simulink model "Project_template_2b"  (R2014b)
settings: Solver=ode23tb  SolverMode=SingleTasking  StartTime=0.0  StopTime=600  RelTol=1e-6  AbsTol=1e-6
values from neighbouring files (symbols this model uses):
  a_0 = 0.6e-05    (= 6e-06)    [Project2B.m]
  A_max_wg = 0.02^2/4*pi    (= 0.000314159265359)    [Project2B.m]
  alpha_REF_manual = 0    [Project2B.m]
  Boost_control = 1    [Project2B.m]
  c_tc_fric = 1e-6    (= 1e-06)    [Project2B.m]
  Cd_wg = 0.9    [Project2B.m]
  dP_thrREF = 10e3    (= 10000)    [Project2B.m]
  J_tc = 1e-5    (= 1e-05)    [Project2B.m]
  KiDriver = 0.05    [Project2B.m]
  KpDriver = 0.8    [Project2B.m]
  KpThr = 1*10^-6    (= 1e-06)    [Project2B.m]
  KpWg = 10e-6    (= 1e-05)    [Project2B.m]
  N_e_manual = 1    [Project2B.m]
  N_e_step = 1    [Project2B.m]
  n_r = 2    [Project2B.m]
  NEND = NINI    (= 2500)    [Project2B.m]
  NeRampInit = 800    [Project2B.m]
  NeSlope = 1    [Project2B.m]
  NINI = 2500    [Project2B.m]
  pedEND = 1    [Project2B.m]
  pedINI = 0.0    (= 0)    [Project2B.m]
  pedPos_manual = 1    [Project2B.m]
  pedST = 30    [Project2B.m]
  T_es = mean(T_es)    [Project2B.m]
  T_ic = mean(T_ic)    [Project2B.m]
  tau_wg = 0.1    [Project2B.m]
  TiThr = 0.1    [Project2B.m]
  TiWg = 5    [Project2B.m]
  TqEvsNe =     [TqEvsNeMAP.mat]
  V_D = n_cyl*V_d    [Project2B.m]
  V_d = B^2/4*pi*s    [Project2B.m]
  V_ic = 10e-3    (= 0.01)    [Project2B.m]
  wg_REF_manual = 0    [Project2B.m]
undefined symbols (not defined in the file or in its folder): a_1, a_2, AFs, alphaEND, alphaINI, alphaST, BSRmax, C_2, C_d, c_fi, c_fr_0, C_P0, C_P1, c_r1, c_r2, cp_air, cp_exh, etaCmax, etaCmin, etaTmax, etaTmin, gamma_air, gamma_exh, k, k0, k1, K_I, K_p, n_0, n_1, n_2, n_cyl, n_ig_ch, NeST, Newton, p_amb, pCref, PiC_at_etaCmax, PsiMax, Q11, Q12, Q22, q_LHV, R_air, r_c, R_exh, Raphson, rComp, rho_air, rTurb, t_0, T_0, T_amb, T_hat_bef_thr, T_hat_im, tau_d_bc, tau_lambda, tau_th, TCref, V_em ... (+10)
libraries: simulink x1
(part 2 of 2)

== system Project_template_2b/Engine/m_dot_ac/n_vol ==
  p_im : Inport
  N : Inport  Port=2
  Constant : Constant  Value=n_0
  Gain : Gain  Gain=n_1
  Gain1 : Gain  Gain=n_2
  Sqrt : Sqrt  SaturateOnIntegerOverflow=on
  Sum of Elements : Sum  Inputs=+++
  n_vol : Outport
  wires:
  Sum of Elements/1 -> n_vol/1
  Constant/1 -> Sum of Elements/1
  p_im/1 -> Sqrt/1
  Sqrt/1 -> Gain/1
  Gain/1 -> Sum of Elements/2
  N/1 -> Gain1/1
  Gain1/1 -> Sum of Elements/3

== system Project_template_2b/ECU/Boost Control/Driver gas pedal interpretation/BMEP_ref -> p_im_ref ==
  In1 : Inport
  Add2 : Sum
  Constant2 : Constant  Value=C_P0
  Gain3 : Gain  Gain=1/C_P1
  Out1 : Outport
  wires:
  Constant2/1 -> Add2/2
  In1/1 -> Add2/1
  Gain3/1 -> Out1/1  "p_im_REF"
  Add2/1 -> Gain3/1

== system Project_template_2b/ECU/Boost Control/Throttle Feed Forward /A_eff_ref ==
  m_dot_air_ref : Inport
  Psi : Inport  Port=2
  p_ic : Inport  Port=3
  Divide1 : Product  Inputs=*/
  Divide2 : Product  Inputs=*/
  Gain : Gain  Gain=sqrt(R_air*T_ic)
  A_eff_ref : Outport
  wires:
  Psi/1 -> Divide1/2
  m_dot_air_ref/1 -> Divide1/1
  Divide1/1 -> Gain/1
  Gain/1 -> Divide2/1
  Divide2/1 -> A_eff_ref/1
  p_ic/1 -> Divide2/2

== system Project_template_2b/ECU/Boost Control/Throttle Feed Forward /Cylinder air flow REF ==
  p_im_REF : Inport
  N [rps] : Inport  Port=2
  Gain : Gain  Gain=n_cyl*V_d/(n_r*R_air*T_hat_im)
  Product : Product  Inputs=3
  Volymetrisk effektivitet : Subsystem
  m_dot_ac_REF : Outport
  wires:
  N [rps]/1 -> Product/3, Volymetrisk effektivitet/2(N)
  p_im_REF/1 -> Product/1, Volymetrisk effektivitet/1(" p_im")
  Product/1 -> Gain/1
  Gain/1 -> m_dot_ac_REF/1
  Volymetrisk effektivitet/1(eta_vol) -> Product/2

== system Project_template_2b/ECU/Boost Control/Throttle Feed Forward /Psi(PI) ==
  PI : Inport
  (g+1)/g : Constant  Value=(gamma_air+1)/gamma_air
  2/g : Constant  Value=2/gamma_air
  2g/(g-1) : Constant  Value=(2*gamma_air)/(gamma_air-1)
  DivZeroProtect : MinMax  Function=max  Inputs=2
  Math Function : Math  Operator=pow  SaturateOnIntegerOverflow=on
  Math Function1 : Math  Operator=pow  SaturateOnIntegerOverflow=on
  MinMax : MinMax  Function=max  Inputs=2
  PI critical (2/(g+1))^(g/(g-1)) : Constant  Value=(2/(gamma_air+1))^(gamma_air/(gamma_air-1))
  Product : Product  RndMeth=Zero
  Sqrt : Sqrt  AlgorithmType=Newton-Raphson  SaturateOnIntegerOverflow=on
  Subtract : Sum  Inputs=+-
  "[0,1]" : Saturate  UpperLimit=1  LowerLimit=0
  eps : Constant  Value=eps
  Psi : Outport
  wires:
  DivZeroProtect/1 -> Psi/1
  eps/1 -> DivZeroProtect/2
  Sqrt/1 -> DivZeroProtect/1  "Psi"
  Product/1 -> Sqrt/1
  2g/(g-1)/1 -> Product/2
  Subtract/1 -> Product/1
  Math Function1/1 -> Subtract/2
  Math Function/1 -> Subtract/1
  "[0,1]"/1 -> MinMax/1
  (g+1)/g/1 -> Math Function1/2
  2/g/1 -> Math Function/2
  MinMax/1 -> Math Function1/1, Math Function/1  "PIlim"
  PI critical (2/(g+1))^(g/(g-1))/1 -> MinMax/2
  PI/1 -> "[0,1]"/1  "PI"

== system Project_template_2b/ECU/Fuel Cont/Air cylinder/n_vol ==
  p_im : Inport
  N : Inport  Port=2
  Constant : Constant  Value=n_0
  Gain : Gain  Gain=n_1
  Gain1 : Gain  Gain=n_2
  Sqrt : Sqrt  SaturateOnIntegerOverflow=on
  Sum of Elements : Sum  Inputs=+++
  n_vol : Outport
  wires:
  Sum of Elements/1 -> n_vol/1
  Constant/1 -> Sum of Elements/1
  p_im/1 -> Sqrt/1
  Sqrt/1 -> Gain/1
  Gain/1 -> Sum of Elements/2
  N/1 -> Gain1/1
  Gain1/1 -> Sum of Elements/3

== system Project_template_2b/Engine/Cylinder/W_ig/eta_tilde_ig ==
  lambda_cyl : Inport
  Constant : Constant
  Gain : Gain  Gain=(1-1/r_c^(gamma_air-1))*n_ig_ch
  MinMax : MinMax  Inputs=2
  eta_tilde_ig : Outport
  wires:
  lambda_cyl/1 -> MinMax/1
  Constant/1 -> MinMax/2
  MinMax/1 -> Gain/1
  Gain/1 -> eta_tilde_ig/1

== system Project_template_2b/Engine/Turbocharger/Compressor/PiCmax ==
  Tamb : Inport
  w_tc : Inport  Port=2
  Add : Sum
  Constant : Constant
  Constant1 : Constant  Value=gamma_air/(gamma_air-1)
  Divide : Product  Inputs=*/
  Gain : Gain  Gain=rComp
  Gain1 : Gain  Gain=PsiMax/(2*cp_air)
  Math Function : Math  Operator=square  SaturateOnIntegerOverflow=on
  Math Function1 : Math  Operator=pow  SaturateOnIntegerOverflow=on
  PiCmax : Outport
  wires:
  Math Function1/1 -> PiCmax/1
  Tamb/1 -> Divide/2
  w_tc/1 -> Gain/1
  Gain/1 -> Math Function/1
  Math Function/1 -> Gain1/1
  Gain1/1 -> Divide/1
  Divide/1 -> Add/1
  Constant/1 -> Add/2
  Add/1 -> Math Function1/1
  Constant1/1 -> Math Function1/2

== system Project_template_2b/Engine/Turbocharger/Compressor/Tc ==
  etaC : Inport
  PiC : Inport  Port=2
  Tamb : Inport  Port=3
  Add : Sum  Inputs=+-
  Add1 : Sum
  Constant : Constant  Value=(gamma_air-1)/gamma_air
  Constant1 : Constant
  Divide : Product  Inputs=*/
  Math Function : Math  Operator=pow  SaturateOnIntegerOverflow=on
  Product : Product
  Tc : Outport
  wires:
  Add1/1 -> Tc/1
  PiC/1 -> Math Function/1
  etaC/1 -> Divide/2
  Tamb/1 -> Add1/2, Product/2
  Constant/1 -> Math Function/2
  Constant1/1 -> Add/2
  Math Function/1 -> Add/1
  Add/1 -> Divide/1
  Divide/1 -> Product/1
  Product/1 -> Add1/1

== system Project_template_2b/Engine/Turbocharger/Compressor/Tq_c ==
  Wc : Inport
  Tc : Inport  Port=2
  Tamb : Inport  Port=3
  w_tc : Inport  Port=4
  Add : Sum  Inputs=+-
  Divide : Product  Inputs=*/
  Gain : Gain  Gain=cp_air
  Product : Product
  Tq_c : Outport
  wires:
  w_tc/1 -> Divide/2
  Wc/1 -> Product/1
  Tc/1 -> Add/1
  Tamb/1 -> Add/2
  Add/1 -> Gain/1
  Gain/1 -> Product/2
  Product/1 -> Divide/1
  Divide/1 -> Tq_c/1

== system Project_template_2b/Engine/Turbocharger/Compressor/WcCorr2Wc ==
  p_amb : Inport
  T_amb : Inport  Port=2
  m_dot_cCorr : Inport  Port=3
  Constant : Constant  Value=0
  Divide : Product  Inputs=*/
  Gain : Gain  Gain=1/TCref
  Gain1 : Gain  Gain=1/pCref
  MinMax : MinMax  Function=max  Inputs=2
  Product : Product
  Sqrt : Sqrt  SaturateOnIntegerOverflow=on
  m_dot_c : Outport
  wires:
  m_dot_cCorr/1 -> Product/1
  p_amb/1 -> Gain1/1
  T_amb/1 -> Gain/1
  Product/1 -> m_dot_c/1
  Gain1/1 -> Divide/1
  Sqrt/1 -> Divide/2
  Divide/1 -> Product/2
  MinMax/1 -> Sqrt/1
  Gain/1 -> MinMax/1
  Constant/1 -> MinMax/2

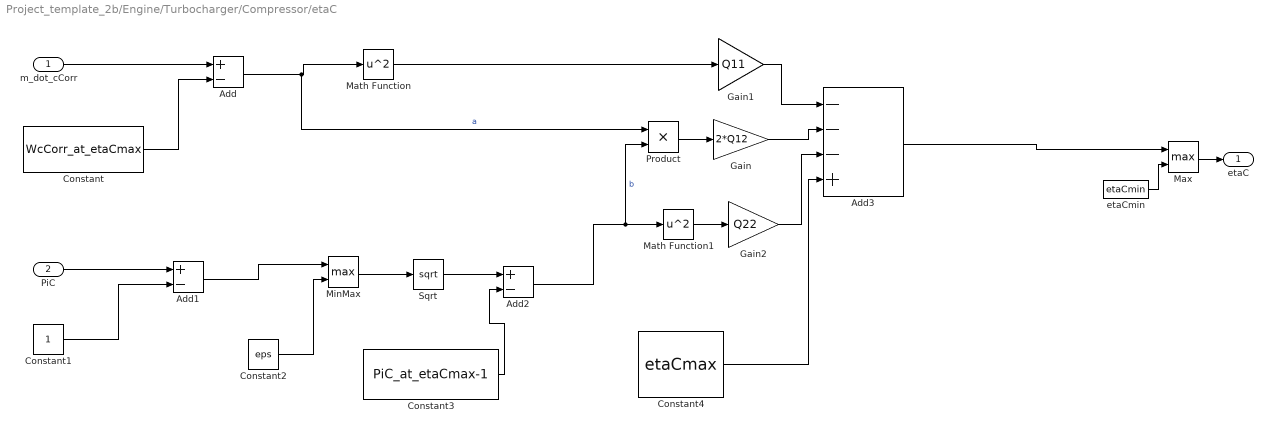
== system Project_template_2b/Engine/Turbocharger/Compressor/etaC ==
  m_dot_cCorr : Inport
  PiC : Inport  Port=2
  Add : Sum  Inputs=+-
  Add1 : Sum  Inputs=+-
  Add2 : Sum  Inputs=+-
  Add3 : Sum  Inputs=---+
  Constant : Constant  Value=WcCorr_at_etaCmax
  Constant1 : Constant
  Constant2 : Constant  Value=eps
  Constant3 : Constant  Value=PiC_at_etaCmax-1
  Constant4 : Constant  Value=etaCmax
  Gain : Gain  Gain=2*Q12
  Gain1 : Gain  Gain=Q11
  Gain2 : Gain  Gain=Q22
  Math Function : Math  Operator=square  SaturateOnIntegerOverflow=on
  Math Function1 : Math  Operator=square  SaturateOnIntegerOverflow=on
  Max : MinMax  Function=max  Inputs=2
  MinMax : MinMax  Function=max  Inputs=2
  Product : Product
  Sqrt : Sqrt  SaturateOnIntegerOverflow=on
  etaCmin : Constant  Value=etaCmin
  etaC : Outport
  wires:
  PiC/1 -> Add1/1
  m_dot_cCorr/1 -> Add/1
  Max/1 -> etaC/1
  etaCmin/1 -> Max/2
  Add3/1 -> Max/1
  Constant/1 -> Add/2
  Add/1 -> Product/1, Math Function/1  "a"
  Constant1/1 -> Add1/2
  Constant2/1 -> MinMax/2
  Add1/1 -> MinMax/1
  MinMax/1 -> Sqrt/1
  Sqrt/1 -> Add2/1
  Constant3/1 -> Add2/2
  Math Function/1 -> Gain1/1
  Gain1/1 -> Add3/1
  Gain/1 -> Add3/2
  Gain2/1 -> Add3/3
  Add2/1 -> Product/2, Math Function1/1  "b"
  Math Function1/1 -> Gain2/1
  Product/1 -> Gain/1
  Constant4/1 -> Add3/4

== system Project_template_2b/Engine/Turbocharger/Compressor/m_dot_cCorr ==
  PiCmax : Inport
  PiC : Inport  Port=2
  Add : Sum  Inputs=-+
  Constant : Constant
  Constant1 : Constant  Value=eps
  Divide : Product  Inputs=/*
  Gain : Gain  Gain=WcCorrMax
  Math Function : Math  Operator=square  SaturateOnIntegerOverflow=on
  MinMax : MinMax  Function=max  Inputs=2
  Sqrt : Sqrt  SaturateOnIntegerOverflow=on
  m_dot_cCorr : Outport
  wires:
  PiC/1 -> Divide/2
  PiCmax/1 -> Divide/1
  Gain/1 -> m_dot_cCorr/1  "m_dot_cCorr"
  Divide/1 -> Math Function/1
  Constant/1 -> Add/2
  Math Function/1 -> Add/1
  Sqrt/1 -> Gain/1
  MinMax/1 -> Sqrt/1
  Add/1 -> MinMax/1
  Constant1/1 -> MinMax/2

== system Project_template_2b/Engine/Turbocharger/Turbine/BSR ==
  T_em : Inport
  PiT : Inport  Port=2
  w_tc [rad/s] : Inport  Port=3
  Add : Sum  Inputs=-+
  Constant : Constant  Value=-(gamma_exh-1)/gamma_exh
  Constant1 : Constant
  Divide : Product  Inputs=*/
  Gain : Gain  Gain=2*cp_exh
  Gain1 : Gain  Gain=rTurb
  Math Function : Math  Operator=pow  SaturateOnIntegerOverflow=on
  Product : Product
  Sqrt : Sqrt  SaturateOnIntegerOverflow=on
  BSR : Outport
  wires:
  PiT/1 -> Math Function/1
  Constant/1 -> Math Function/2
  Math Function/1 -> Add/1
  Constant1/1 -> Add/2
  Add/1 -> Product/1
  T_em/1 -> Product/2
  Product/1 -> Gain/1
  Sqrt/1 -> Divide/2
  Gain1/1 -> Divide/1
  w_tc [rad/s]/1 -> Gain1/1
  Divide/1 -> BSR/1
  Gain/1 -> Sqrt/1

== system Project_template_2b/Engine/Turbocharger/Turbine/PiT ==
  p_em : Inport
  p_t : Inport  Port=2
  MinMax : MinMax  Function=max  Inputs=2
  Product4 : Product  Inputs=*/  RndMeth=Zero
  one1 : Constant
  PiT : Outport
  wires:
  p_t/1 -> Product4/2
  MinMax/1 -> PiT/1  "PiT"
  p_em/1 -> Product4/1
  one1/1 -> MinMax/2
  Product4/1 -> MinMax/1

== system Project_template_2b/Engine/Turbocharger/Turbine/TFP2Wt ==
  p_em [Pa] : Inport
  TFP : Inport  Port=2
  T_em : Inport  Port=3
  Constant1 : Constant  Value=1e-3
  Divide : Product  Inputs=*/
  Product : Product  Inputs=3
  Sqrt : Sqrt  SaturateOnIntegerOverflow=on
  Wt : Outport
  wires:
  Divide/1 -> Wt/1
  TFP/1 -> Product/1
  p_em [Pa]/1 -> Product/2
  Product/1 -> Divide/1
  T_em/1 -> Sqrt/1
  Sqrt/1 -> Divide/2
  Constant1/1 -> Product/3

== system Project_template_2b/Engine/Turbocharger/Turbine/TFPmod ==
  PiT : Inport
  Add : Sum  Inputs=-+
  Constant : Constant  Value=-k1
  Constant1 : Constant
  Constant2 : Constant  Value=eps
  Gain : Gain  Gain=k0
  Math Function : Math  Operator=pow  SaturateOnIntegerOverflow=on
  MinMax : MinMax  Function=max  Inputs=2
  Sqrt : Sqrt  SaturateOnIntegerOverflow=on
  TFPmod : Outport
  wires:
  PiT/1 -> Math Function/1
  Constant/1 -> Math Function/2
  Math Function/1 -> Add/1
  Constant1/1 -> Add/2
  Constant2/1 -> MinMax/2
  Add/1 -> MinMax/1
  MinMax/1 -> Sqrt/1
  Sqrt/1 -> Gain/1
  Gain/1 -> TFPmod/1

== system Project_template_2b/Engine/Turbocharger/Turbine/Tq_t ==
  Wt : Inport
  Tem : Inport  Port=2
  Tt : Inport  Port=3
  w_tc : Inport  Port=4
  Add : Sum  Inputs=+-
  Divide : Product  Inputs=*/
  Gain : Gain  Gain=cp_exh
  Product : Product
  Tq_t : Outport
  wires:
  Tt/1 -> Add/2
  Tem/1 -> Add/1
  Add/1 -> Gain/1
  Gain/1 -> Product/2
  Wt/1 -> Product/1
  w_tc/1 -> Divide/2
  Product/1 -> Divide/1
  Divide/1 -> Tq_t/1

== system Project_template_2b/Engine/Turbocharger/Turbine/Tt ==
  Tem : Inport
  etaT : Inport  Port=2
  PiT : Inport  Port=3
  Add : Sum  Inputs=-+
  Add1 : Sum  Inputs=+-
  Constant : Constant  Value=-(gamma_exh-1)/gamma_exh
  Constant1 : Constant
  Constant2 : Constant
  Math Function : Math  Operator=pow  SaturateOnIntegerOverflow=on
  Product : Product
  Product1 : Product
  Tt : Outport
  wires:
  PiT/1 -> Math Function/1
  Constant/1 -> Math Function/2
  Constant1/1 -> Add/2
  Add/1 -> Product/1
  etaT/1 -> Product1/2
  Tem/1 -> Product/2
  Product/1 -> Tt/1
  Product1/1 -> Add/1
  Constant2/1 -> Add1/1
  Math Function/1 -> Add1/2
  Add1/1 -> Product1/1

== system Project_template_2b/Engine/Turbocharger/Turbine/etaT ==
  BSR : Inport
  Add : Sum  Inputs=+-
  Add1 : Sum  Inputs=-+
  Constant : Constant  Value=BSRmax
  Constant1 : Constant
  Divide : Product  Inputs=*/
  Gain : Gain  Gain=etaTmax
  Math Function : Math  Operator=square  SaturateOnIntegerOverflow=on
  Max : MinMax  Function=max  Inputs=2
  etaTmin : Constant  Value=etaTmin
  etaT : Outport
  wires:
  etaTmin/1 -> Max/2
  Max/1 -> etaT/1
  BSR/1 -> Add/1
  Constant/1 -> Divide/2, Add/2
  Add/1 -> Divide/1
  Divide/1 -> Math Function/1
  Math Function/1 -> Add1/1
  Constant1/1 -> Add1/2
  Add1/1 -> Gain/1
  Gain/1 -> Max/1

== system Project_template_2b/Engine/Turbocharger/Wastegate/Psi(PI) ==
  PI : Inport
  (g+1)/g : Constant  Value=(gamma_air+1)/gamma_air
  2/g : Constant  Value=2/gamma_air
  2g/(g-1) : Constant  Value=(2*gamma_air)/(gamma_air-1)
  Math Function : Math  Operator=pow  SaturateOnIntegerOverflow=on
  Math Function1 : Math  Operator=pow  SaturateOnIntegerOverflow=on
  MinMax : MinMax  Function=max  Inputs=2
  PI critical (2/(g+1))^(g/(g-1)) : Constant  Value=(2/(gamma_air+1))^(gamma_air/(gamma_air-1))
  Product : Product  RndMeth=Zero
  Sqrt : Sqrt  AlgorithmType=Newton-Raphson  SaturateOnIntegerOverflow=on
  Subtract : Sum  Inputs=+-
  "[0, 1]" : Saturate  UpperLimit=1  LowerLimit=0
  Psi : Outport
  wires:
  Sqrt/1 -> Psi/1  "Psi"
  Product/1 -> Sqrt/1
  2g/(g-1)/1 -> Product/2
  Subtract/1 -> Product/1
  Math Function1/1 -> Subtract/2
  Math Function/1 -> Subtract/1
  "[0, 1]"/1 -> MinMax/1
  (g+1)/g/1 -> Math Function1/2
  2/g/1 -> Math Function/2
  MinMax/1 -> Math Function1/1, Math Function/1  "PIlim"
  PI critical (2/(g+1))^(g/(g-1))/1 -> MinMax/2
  PI/1 -> "[0, 1]"/1  "PI"

== system Project_template_2b/ECU/Boost Control/Throttle Feed Forward /Cylinder air flow REF/Volymetrisk effektivitet ==
  " p_im" : Inport
  N : Inport  Port=2
  Constant : Constant  Value=n_0
  Gain : Gain  Gain=n_1
  Gain1 : Gain  Gain=n_2
  Sqrt : Sqrt  SaturateOnIntegerOverflow=on
  Sum of Elements : Sum  Inputs=+++
  eta_vol : Outport
  wires:
  Sum of Elements/1 -> eta_vol/1
  Constant/1 -> Sum of Elements/1
  " p_im"/1 -> Sqrt/1
  Sqrt/1 -> Gain/1
  Gain/1 -> Sum of Elements/2
  N/1 -> Gain1/1
  Gain1/1 -> Sum of Elements/3
